simulink model "WormAndGearConstraint0x5B10x5D"  (R2024a)
settings: Solver=ode45  StartTime=0.0  StopTime=20  MaxStep=0.01  RelTol=1e-3
PreLoadFcn:
  | addpath(fullfile('WormAndGearConstraintSupport','Data'));
  | addpath(fullfile('WormAndGearConstraintSupport','Scripts'));
model workspace: external: MATLAB File WormAndGearConstraintParameters.m (data not in the file)
undefined symbols (not defined in the file): driveconn, frame, framemount, slewdrive, solarpanel, support, X, Y, Z
libraries: sm_lib x393, nesl_utility x10, fl_lib x4, SignalEditorBlockLib x2, fl_ps_legacy_lib x1
(part 1 of 11)
CloseFcn:
  | rmpath(fullfile('WormAndGearConstraintSupport','Data'));
  | rmpath(fullfile('WormAndGearConstraintSupport','Scripts'));
Description:
  | Using the Worm and Gear Constraint Block - Solar Tracker
settings Model: Creator=The MathWorks, Inc.  LastModifiedBy=Abhilash LN
settings SolverCC: AlgebraicLoopSolver=TrustRegion
settings OptimizationCC: ReuseModelBlockBuffer=off
settings DebuggingCC: UnconnectedInputMsg=warning  UnconnectedOutputMsg=warning  UnconnectedLineMsg=warning  SubsystemReferenceDiagnosticForUnitTest=warning  ArithmeticOperatorsInVariantConditions=warning
settings ModelReferenceCC: EnableRefExpFcnMdlSchedulingChecks=on
settings SFSimCC: SimUseLocalCustomCode=off  CustomCodeUndefinedFunction=UseInterfaceOnly
settings RTWCC: RTWUseLocalCustomCode=off  GPUComputeCapability=3.5
settings CodeAppCC: StateflowObjectComments=on
settings ConfigComp: CovMetricSettings=dswe
settings SimscapeCC: SimscapeNormalizeSystem=off  SimscapeNominalValues="[{\"value\":\"10\",\"unit\":\"V\"},{\"value\":\"1\",\"unit\":\"A\"},{\"value\":\"10\",\"unit\":\"N*m\"},{\"value\":\"10\",\"unit\":\"bar\"},{\"value\":\"100\",\"unit\":\"kJ/kg\"},{\"value\":\"1\",\"unit\":\"kW\"},{\"value\":\"300\",\"unit\":\"K\"},{\"value\":\"100\",\"unit\":\"cm^3/s\"},{\"value\":\"1\",\"unit\":\"kN\"},{\"value\":\"1\",\"unit\":\"g/cm^3\"},{\"value\":\"1\",\"unit\":\"l\"},{\"value\":\"1\",\"unit\":\"cm^2\"},{\"value\":\"60\",\"unit\":\"Hz\"}]"  SimscapeLogType=all  SimscapeLogSimulationStatistics=on  SimscapeLogName=simlogWormAndGearConstraint
settings DiagnosticsConfigSet: SimMechanicsUnconnectedFramePorts=none
settings ExplorerConfigSet: InternalSimMechanicsExplorerSettings="<ExplorerConfiguration><canonicalview>default</canonicalview><AnimationSetting><BasePlaybackSpeed>1.0</BasePlaybackSpeed><PlaybackSpeedFactor>1.0</PlaybackSpeedFactor></AnimationSetting><TilePanel><TileInfo><Tiles Columns=\"1\" Count=\"2\" Rows=\"2\"><Column Left=\"2\" Weight=\"1\"/><Column Left=\"959\" Weight=\"0.5003\"/><Row Top=\"2\" Weight=\"0.499\"/><Row Top=\"438\" Weight=\"0.501\"/><Row Top=\"875\"/><Tile Height=\"1\" Width=\"1\" X=\"0\" Y=\"0\"/><Tile Height=\"1\" Width=\"1\" X=\"0\" Y=\"1\"/></Tiles></TileInfo><SceneInfo><SceneViewer><BGColor><R>0.60000002384185791</R><G>0.60000002384185791</G><B>0.60000002384185791</B></BGColor><Camera><DoPerspective>off</DoPerspective><Position><X>1.5722270375482781</X><Y>0.036026125950558319</Y><Z>2.5132450829803226</Z></Position><Center><X>0.030597625568977493</X><Y>1.5776555379298589</Y><Z>0.97161567100102131</Z></Center><Up><X>-0.40824829046386307</X><Y>0.40824829046386307</Y><Z>0.81649658092772615</Z></Up><ViewLimDist>1</ViewLimDist><YLim>1.5517509961128235</YLim><XLim>3.445105256006924</XLim></Camera></SceneViewer><SceneViewer><BGColor><R>0.60000002384185791</R><G>0.60000002384185791</G><B>0.60000002384185791</B></BGColor><Camera><DoPerspective>on</DoPerspective><Position><X>0.052898448769590822</X><Y>3.2815089600888423</Y><Z>1.0106868675116196</Z></Position><Center><X>-0.01109217435380673</X><Y>3.0487464713239714</Y><Z>0.94979470185928261</Z></Center><Up><X>-0.054323829999052796</X><Y>-0.23871114009518463</Y><Z>0.96956996296744424</Z></Up><ViewLimDist>1</ViewLimDist><YLim>0.46630765815499858</YLim><XLim>1.0328496727358381</XLim></Camera></SceneViewer></SceneInfo></TilePanel><MechEditorPanel><Cameras><Camera><Id>Camera1</Id><Value><Name>Slew Drive View</Name><NativeCamera><PositionKeyframeSet><Keyframe><Time>+0.0000000000000000e+00</Time><Value><X>+5.2898448769590822e-02</X><Y>+3.2815089600888423e+00</Y><Z>+1.0106868675116196e+00</Z></Value></Keyframe></PositionKeyframeSet><CenterKeyframeSet><Keyframe><Time>+0.0000000000000000e+00</Time><Value><X>-1.1092174353806730e-02</X><Y>+3.0487464713239714e+00</Y><Z>+9.4979470185928261e-01</Z></Value></Keyframe></CenterKeyframeSet><UpVectorKeyframeSet><Keyframe><Time>+0.0000000000000000e+00</Time><Value><X>-5.4323829999052796e-02</X><Y>-2.3871114009518463e-01</Y><Z>+9.6956996296744424e-01</Z></Value></Keyframe></UpVectorKeyframeSet></NativeCamera></Value></Camera></Cameras><GfxPanelCameraMap><MapElement CameraMLId=\"Camera1\" GfxPanelIndex=\"1\"/></GfxPanelCameraMap><VideoCreator><PlaybackSpeedRatio>1.0</PlaybackSpeedRatio><FrameRate>30</FrameRate><VideoFormat>Motion JPEG AVI</VideoFormat><FrameSize>auto</FrameSize></VideoCreator></MechEditorPanel></ExplorerConfiguration>"

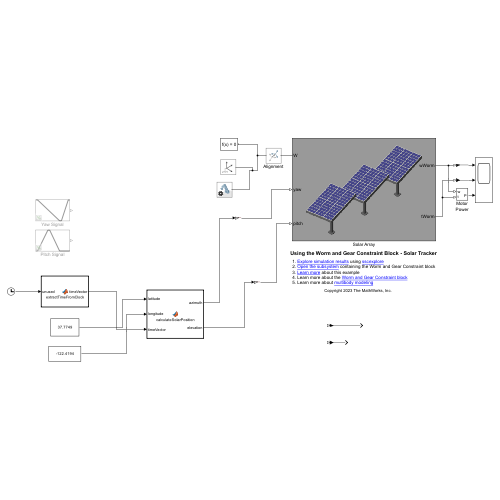
[thumbnail: Simulink's stored preview of the top-level diagram]
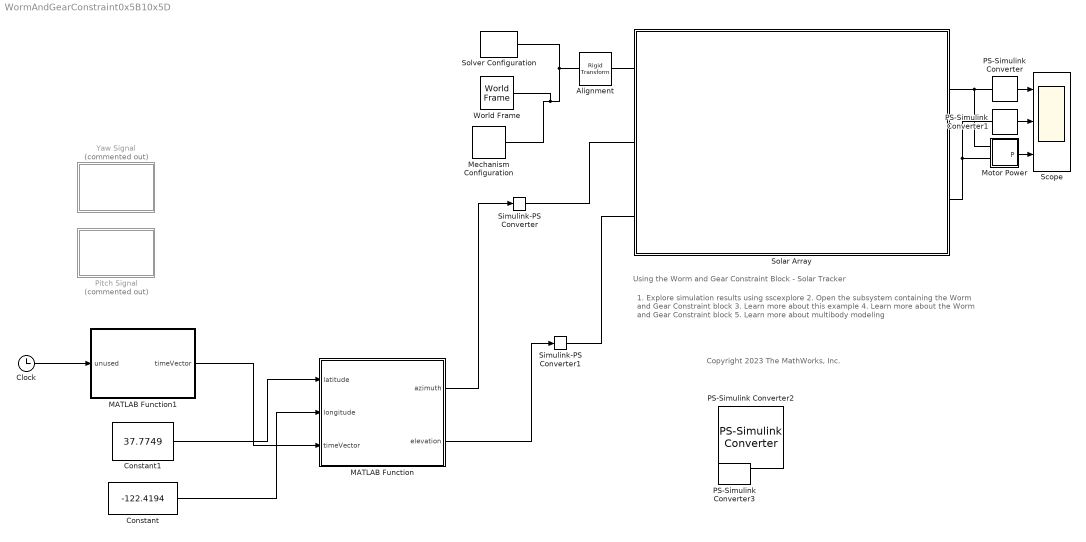
== system WormAndGearConstraint0x5B10x5D ==
  note: Copyright 2023 The MathWorks, Inc.
  note: Using the Worm and Gear Constraint Block - Solar Tracker
  note: 1. Explore simulation results using sscexplore
      | 2. Open the subsystem containing the Worm and Gear Constraint block
      | 3. Learn more about this example
      | 4. Learn more about the Worm and Gear Constraint block
      | 5. Learn more about multibody modeling
  Alignment : sm_lib/Frames and Transforms/Rigid Transform  RotationMethod=AlignedAxes  FollAlignAxisA=+Z  BaseAlignAxisA=+Z  FollAlignAxisB=+Y  BaseAlignAxisB=-X  RotationStandardAxis=+Z  RotationAngle=0.0  RotationAngleUnits=deg  RotationArbitraryAxis=[0 0 1]  RotationSequenceAxes=FollowerAxes  RotationSequence=XYX  RotationSequenceAngles=[0 0 0]  RotationSequenceAnglesUnits=deg  RotationMatrix=[1 0 0; 0 1 0; 0 0 1]  Quaternion=[1 0 0 0]  TranslationMethod=None  TranslationCartesianOffset=[0 0 0]  TranslationCartesianOffsetUnits=m  TranslationStandardAxis=+Z  TranslationStandardOffset=0  TranslationStandardOffsetUnits=m  TranslationROffset=0  TranslationROffsetUnits=m  TranslationThetaOffset=0  TranslationThetaOffsetUnits=deg  TranslationZOffset=0  TranslationZOffsetUnits=m
  Clock : Clock
  Constant : Constant  Value=-122.4194
  Constant1 : Constant  Value=37.7749
  MATLAB Function : MATLAB Function  TreatAsAtomicUnit=on
  MATLAB Function1 : MATLAB Function  TreatAsAtomicUnit=on
  Mechanism Configuration : sm_lib/Utilities/Mechanism Configuration  UniformGravity=Constant  GravityVector=[0 0 -9.80665]  GravityVectorUnits=m/s^2  LinearizationDelta=0.001  JointModeTransitionNonlinearIterations=2
  Motor Power : Subsystem
  PS-Simulink Converter : nesl_utility/PS-Simulink Converter  PhysicalDomain=network_engine_domain  SubClassName=ps_output  LeftPortType=input  RightPortType=output  PseudoPeriodic=off  Frequencies=[]  VectorFormat=1-D array  Unit=deg/s  AffineConversion=off
  PS-Simulink Converter1 : nesl_utility/PS-Simulink Converter  PhysicalDomain=network_engine_domain  SubClassName=ps_output  LeftPortType=input  RightPortType=output  PseudoPeriodic=off  Frequencies=[]  VectorFormat=1-D array  Unit=N*m  AffineConversion=off
  PS-Simulink Converter2 : nesl_utility/PS-Simulink Converter  PhysicalDomain=network_engine_domain  SubClassName=ps_output  LeftPortType=input  RightPortType=output  PseudoPeriodic=off  Frequencies=[]  VectorFormat=inherit  Unit=deg  AffineConversion=off
  PS-Simulink Converter3 : nesl_utility/PS-Simulink Converter  PhysicalDomain=network_engine_domain  SubClassName=ps_output  LeftPortType=input  RightPortType=output  PseudoPeriodic=off  Frequencies=[]  VectorFormat=inherit  Unit=deg  AffineConversion=off
  Pitch Signal : Subsystem  Commented=on
      mask Display: plot([0 1 7 8 14 20],[0 0 1 1 0 0])
  Scope : Scope  NumInputPorts=3
  Simulink-PS Converter : nesl_utility/Simulink-PS Converter  PhysicalDomain=network_engine_domain  SubClassName=ps_input  LeftPortType=input  RightPortType=output  PseudoPeriodic=off  Frequencies=[]  NoiseDistribution=none  NoiseParameters=[]  Unit=1  AffineConversion=off  FilteringAndDerivatives=provide  SimscapeFilterOrder=1  InputFilterTimeConstant=0.001  UdotUserProvided=0
  Simulink-PS Converter1 : nesl_utility/Simulink-PS Converter  PhysicalDomain=network_engine_domain  SubClassName=ps_input  LeftPortType=input  RightPortType=output  PseudoPeriodic=off  Frequencies=[]  NoiseDistribution=none  NoiseParameters=[]  Unit=1  AffineConversion=off  FilteringAndDerivatives=provide  SimscapeFilterOrder=1  InputFilterTimeConstant=0.001  UdotUserProvided=0
  Solar Array : Subsystem
      mask Display:
      | image(fullfile('WormAndGearConstraintSupport','Images','SolarArray.png'));
      | port_label('lconn',1,'W');
      | port_label('lconn',2,'yaw');
      | port_label('lconn',3,'pitch');
      | port_label('rconn',1,'wWorm');
      | port_label('rconn',2,'tWorm');
  Solver Configuration : nesl_utility/Solver Configuration  PhysicalDomain=network_engine_domain  SubClassName=solver  LeftPortType=input  RightPortType=generic  Tones=[]  Harmonics=[]  SimulateNoise=off  Profile=off  UseLocalSampling=off  EnableSwitchedLinearOptims=on  FrequencyDomain=off  UseCCode=off  RelTol=0.001  AbsTol=1e-06  MinStep=1e-09  ToWorkspace=off  RevertToSquareIcSolve=off  NumHomotopyIterations=100  PhasorMode=off  PhasorModeNumHarmonics=1  ConsistencySolver=NEWTON_XTOL_AFTER_FTOL  IndexReductionMethod=DerivativeReplacement  DoDC=off  ResidualTolerance=1e-09  ConsistencyTolSource=GLOBAL  ConsistencyAbsTol=0.001  ConsistencyRelTol=0.001  ConsistencyTolFactor=0.001  UseLocalSolver=off  LocalSolverChoice=NE_BACKWARD_EULER_ADVANCER  ResolveIndetEquations=on  FunctionEvalNumThread=1  LocalSolverSampleTime=0.001  DoFixedCost=off  MaxNonlinIter=3  MaxModeIter=2  ComputeImpulses=off  ImpulseIterations=2  LinearAlgebra=Sparse  LinearAlgebraNumThread=0  EquationFormulation=NE_TIME_EF  DelaysMemoryBudget=1024  AutomaticFiltering=on  FilteringTimeConstant=0.001  PartitionStorageMethod=AS_NEEDED  PartitionMemoryBudget=1024  PartitionMethod=FAST  MultibodyUseLocalSolver=off  MultibodyLocalSolverChoice=ODE1  MultibodyLocalSolverSampleTime=0.001
  World Frame : sm_lib/Frames and Transforms/World Frame
  Yaw Signal : Subsystem  Commented=on
      mask Display: plot([0 1 14 15 19 20], [0 0 -1 -1 0 0])
  wires:
  PS-Simulink Converter1/1 -> Scope/2
  PS-Simulink Converter/1 -> Scope/1
  Motor Power/1(P) -> Scope/3
  Constant/1 -> MATLAB Function/2(longitude)
  MATLAB Function1/1(timeVector) -> MATLAB Function/3(timeVector)
  Clock/1 -> MATLAB Function1/1(unused)
  Constant1/1 -> MATLAB Function/1(latitude)
  MATLAB Function/2(elevation) -> Simulink-PS Converter1/1
  MATLAB Function/1(azimuth) -> Simulink-PS Converter/1
  connections:
  World Frame/RConn1 -- Solver Configuration/RConn1 -- Alignment/LConn1 -- Mechanism Configuration/RConn1
  Alignment/RConn1 -- Solar Array/LConn1
  PS-Simulink Converter/LConn1 -- Motor Power/LConn1 -- Solar Array/RConn1
  PS-Simulink Converter1/LConn1 -- Motor Power/LConn2 -- Solar Array/RConn2
  Simulink-PS Converter/RConn1 -- Solar Array/LConn2
  Simulink-PS Converter1/RConn1 -- Solar Array/LConn3

== system WormAndGearConstraint0x5B10x5D/Motor Power ==
  Motor Power : fl_ps_legacy_lib/Legacy Physical Signals/Functions/PS Product
  PS-Simulink Converter2 : nesl_utility/PS-Simulink Converter  PhysicalDomain=network_engine_domain  SubClassName=ps_output  LeftPortType=input  RightPortType=output  PseudoPeriodic=off  Frequencies=[]  VectorFormat=1-D array  Unit=kW  AffineConversion=off
  w : PMIOPort  Side=Left
  t : PMIOPort  Port=2  Side=Left
  P : Outport
  wires:
  PS-Simulink Converter2/1 -> P/1
  connections:
  PS-Simulink Converter2/LConn1 -- Motor Power/RConn1
  Motor Power/LConn2 -- t/RConn1
  Motor Power/LConn1 -- w/RConn1

== system WormAndGearConstraint0x5B10x5D/Pitch Signal ==
  Pitch Signal : SignalEditorBlockLib/Signal Editor  FileName=WormAndGearConstraintInput2.mat  ActiveScenario=Group_1  ActiveSignal=Signal 2  IsBus=off  OutputBusObjectStr=Bus: BusObject  SampleTime=0  OutputAfterFinalValue=Extrapolation  Unit=inherit  PreserveSignalName=on  ApplySigPropsToAllScenarios=on  ApplySigPropsToAllSignals=off
  Simulink-PS Converter2 : nesl_utility/Simulink-PS Converter  PhysicalDomain=network_engine_domain  SubClassName=ps_input  LeftPortType=input  RightPortType=output  PseudoPeriodic=off  Frequencies=[]  NoiseDistribution=none  NoiseParameters=[]  Unit=deg  AffineConversion=off  FilteringAndDerivatives=filter  SimscapeFilterOrder=2  InputFilterTimeConstant=pitchsignal.t_c  UdotUserProvided=1
  Signal : PMIOPort  Side=Right
  wires:
  Pitch Signal/1 -> Simulink-PS Converter2/1
  connections:
  Signal/RConn1 -- Simulink-PS Converter2/RConn1

== system WormAndGearConstraint0x5B10x5D/Solar Array ==
  Solar Tracker1 : Subsystem
      mask Display:
      | image(fullfile('WormAndGearConstraintSupport','Images','SolarTracker.png'));
      | port_label('lconn',1,'B');
      | port_label('lconn',2,'y');
      | port_label('lconn',3,'p');
  Solar Tracker2 : Subsystem
      mask Display:
      | image(fullfile('WormAndGearConstraintSupport','Images','SolarTracker.png'));
      | port_label('lconn',1,'B');
      | port_label('lconn',2,'y');
      | port_label('lconn',3,'p');
  Solar Tracker3 : Subsystem
      mask Display:
      | image(fullfile('WormAndGearConstraintSupport','Images','SolarTracker.png'));
      | port_label('lconn',1,'B');
      | port_label('lconn',2,'y');
      | port_label('lconn',3,'p');
      | port_label('rconn',1,'w');
      | port_label('rconn',2,'t');
  Tracker1 xForm : sm_lib/Frames and Transforms/Rigid Transform  RotationMethod=None  FollAlignAxisA=+X  BaseAlignAxisA=+Y  FollAlignAxisB=+Y  BaseAlignAxisB=+Z  RotationStandardAxis=+Z  RotationAngle=0.0  RotationAngleUnits=deg  RotationArbitraryAxis=[0 0 1]  RotationSequenceAxes=FollowerAxes  RotationSequence=XYX  RotationSequenceAngles=[0 0 0]  RotationSequenceAnglesUnits=deg  RotationMatrix=[1 0 0; 0 1 0; 0 0 1]  Quaternion=[1 0 0 0]  TranslationMethod=Cartesian  TranslationCartesianOffset=tracker1_offset  TranslationCartesianOffsetUnits=m  TranslationStandardAxis=+Z  TranslationStandardOffset=0  TranslationStandardOffsetUnits=m  TranslationROffset=0  TranslationROffsetUnits=m  TranslationThetaOffset=0  TranslationThetaOffsetUnits=deg  TranslationZOffset=0  TranslationZOffsetUnits=m
  Tracker2 xForm : sm_lib/Frames and Transforms/Rigid Transform  RotationMethod=None  FollAlignAxisA=+Z  BaseAlignAxisA=+Z  FollAlignAxisB=+Y  BaseAlignAxisB=-X  RotationStandardAxis=+Z  RotationAngle=0.0  RotationAngleUnits=deg  RotationArbitraryAxis=[0 0 1]  RotationSequenceAxes=FollowerAxes  RotationSequence=XYX  RotationSequenceAngles=[0 0 0]  RotationSequenceAnglesUnits=deg  RotationMatrix=[1 0 0; 0 1 0; 0 0 1]  Quaternion=[1 0 0 0]  TranslationMethod=Cartesian  TranslationCartesianOffset=tracker2_offset  TranslationCartesianOffsetUnits=m  TranslationStandardAxis=+Z  TranslationStandardOffset=0  TranslationStandardOffsetUnits=m  TranslationROffset=0  TranslationROffsetUnits=m  TranslationThetaOffset=0  TranslationThetaOffsetUnits=deg  TranslationZOffset=0  TranslationZOffsetUnits=m
  Tracker3 xForm : sm_lib/Frames and Transforms/Rigid Transform  RotationMethod=None  FollAlignAxisA=+X  BaseAlignAxisA=+Y  FollAlignAxisB=+Y  BaseAlignAxisB=+Z  RotationStandardAxis=+Z  RotationAngle=0.0  RotationAngleUnits=deg  RotationArbitraryAxis=[0 0 1]  RotationSequenceAxes=FollowerAxes  RotationSequence=XYX  RotationSequenceAngles=[0 0 0]  RotationSequenceAnglesUnits=deg  RotationMatrix=[1 0 0; 0 1 0; 0 0 1]  Quaternion=[1 0 0 0]  TranslationMethod=Cartesian  TranslationCartesianOffset=tracker3_offset  TranslationCartesianOffsetUnits=m  TranslationStandardAxis=+Z  TranslationStandardOffset=0  TranslationStandardOffsetUnits=m  TranslationROffset=0  TranslationROffsetUnits=m  TranslationThetaOffset=0  TranslationThetaOffsetUnits=deg  TranslationZOffset=0  TranslationZOffsetUnits=m
  W : PMIOPort  Side=Left
  wWorm : PMIOPort  Port=2  Side=Right
  yaw : PMIOPort  Port=3  Side=Left
  tWorm : PMIOPort  Port=4  Side=Right
  pitch : PMIOPort  Port=5  Side=Left
  connections:
  Tracker3 xForm/LConn1 -- Tracker1 xForm/LConn1 -- W/RConn1 -- Tracker2 xForm/LConn1
  Tracker3 xForm/RConn1 -- Solar Tracker3/LConn1
  Solar Tracker3/RConn2 -- tWorm/RConn1
  Solar Tracker3/LConn3 -- Solar Tracker2/LConn3 -- Solar Tracker1/LConn3 -- pitch/RConn1
  Solar Tracker3/RConn1 -- wWorm/RConn1
  Solar Tracker2/LConn2 -- Solar Tracker1/LConn2 -- Solar Tracker3/LConn2 -- yaw/RConn1
  Tracker2 xForm/RConn1 -- Solar Tracker2/LConn1
  Tracker1 xForm/RConn1 -- Solar Tracker1/LConn1

== system WormAndGearConstraint0x5B10x5D/Yaw Signal ==
  Simulink-PS Converter1 : nesl_utility/Simulink-PS Converter  PhysicalDomain=network_engine_domain  SubClassName=ps_input  LeftPortType=input  RightPortType=output  PseudoPeriodic=off  Frequencies=[]  NoiseDistribution=none  NoiseParameters=[]  Unit=deg  AffineConversion=off  FilteringAndDerivatives=filter  SimscapeFilterOrder=2  InputFilterTimeConstant=yawsignal.t_c  UdotUserProvided=1
  Yaw Signal : SignalEditorBlockLib/Signal Editor  FileName=WormAndGearConstraintInput1.mat  ActiveScenario=Group_1  ActiveSignal=Signal  IsBus=off  OutputBusObjectStr=Bus: BusObject  SampleTime=0  Interpolate=off  ZeroCross=off  OutputAfterFinalValue=Setting to zero  Unit=inherit  PreserveSignalName=on  ApplySigPropsToAllScenarios=on  ApplySigPropsToAllSignals=off
  Signal : PMIOPort  Side=Right
  wires:
  Yaw Signal/1 -> Simulink-PS Converter1/1
  connections:
  Signal/RConn1 -- Simulink-PS Converter1/RConn1

== system WormAndGearConstraint0x5B10x5D/Solar Array/Solar Tracker1 ==
  Drive Connection : Subsystem  AncestorBlock=WormAndGearConstraintLibrary/Drive Connection  mask(Drive Connection){connRadius=driveconn.connectionRadius, connThickness=driveconn.connectionThickness, connLength=driveconn.connectionLength, bracketWidth=driveconn.bracketWidthHeight, bracketThickness=driveconn.bracketThickness, holeRadius=driveconn.holeRadius, holeOffset=driveconn.holeOffset, baseThickness=driveconn.baseThickness, rho=driveconn.density, color=driveconn.color}
      mask prompts: connRadius "Connection Radius (m)"; connThickness "Connection Thickness (m)"; connLength "Connection Length (m)"; bracketWidth "Bracket Width and Height (m)"; bracketThickness "Bracket Thickness (m)"; holeRadius "Hole Radius (m)"; holeOffset "Hole Offset (m)"; baseThickness "Base Thickness (m)"; rho "Density (kg/m^3)"; color "Color [r g b]"
      mask help:
      | This block models the element that connects the solar array assembly to the slew drive.
      |
      | Port B corresponds to the center of the base face of the drive connection. Port H corresponds to the center of the bracket hole.
      mask init:
      | baseAngle = atan(bracketWidth / bracketThickness);
      | baseRadius = 0.5 * bracketThickness / cos(baseAngle);
      settings: LibrarySourceBlock=sm_solar_tracker_lib/Drive Connection
      mask DialogControl Tab1 Prompt: Dimensions
      mask DialogControl Tab2 Prompt: Material Properties
      mask Display:
      | image(fullfile('WormAndGearConstraintSupport','Images','DriveConnection.png'));
      | port_label('lconn',1,'B');
      | port_label('rconn',1,'H');
  PS Terminator : fl_lib/Physical Signals/Sinks/PS Terminator
  PS Terminator1 : fl_lib/Physical Signals/Sinks/PS Terminator
  Panel Revolute : sm_lib/Joints/Revolute Joint  JointMode=Normal  CompositeWrenchDir=FollowerOnBase  CompositeWrenchFrame=BaseFrame  SenseConstraintForce=off  SenseConstraintTorque=off  SenseTotalForce=off  SenseTotalTorque=off  PositionTargetSpecify=on  PositionTargetPriority=High  PositionTargetValue=panelrevolute.q0  PositionTargetValueUnits=deg  VelocityTargetSpecify=off  VelocityTargetPriority=High  VelocityTargetValue=0  VelocityTargetValueUnits=deg/s  EquilibriumPosition=0  EquilibriumPositionUnits=deg  SpringStiffness=0  SpringStiffnessUnits=N*m/deg  DampingCoefficient=0  DampingCoefficientUnits=N*m/(deg/s)  LowerLimitSpecify=off  LowerLimitBound=-90  LowerLimitBoundUnits=deg  LowerLimitStiffness=1e4  LowerLimitStiffnessUnits=N*m/deg  LowerLimitDamping=10  LowerLimitDampingUnits=N*m/(deg/s)  LowerLimitTransitionRegionWidth=0.1  LowerLimitTransitionRegionWidthUnits=deg  UpperLimitSpecify=off  UpperLimitBound=90  UpperLimitBoundUnits=deg  UpperLimitStiffness=1e4  UpperLimitStiffnessUnits=N*m/deg  UpperLimitDamping=10  UpperLimitDampingUnits=N*m/(deg/s)  UpperLimitTransitionRegionWidth=0.1  UpperLimitTransitionRegionWidthUnits=deg  TorqueActuationMode=ComputedTorque  MotionActuationMode=InputMotion  SensePosition=off  SenseVelocity=off  SenseAcceleration=off  SenseTorqueForce=off  SenseLowerLimitTorqueForce=off  SenseUpperLimitTorqueForce=off
  Slew Drive : Subsystem  AncestorBlock=WormAndGearConstraintLibrary/Slew Drive  mask(Slew Drive){wormLeadAngle=slewdrive.wormLeadAngle, wormLength=slewdrive.wormLength, gearOuterRadius=slewdrive.gearOuterRadius, gearInnerRadius=slewdrive.gearInnerRadius, gearExposedRadius=slewdrive.gearExposedRadius, ratio=slewdrive.ratio, housingThickness=slewdrive.housingThickness, bWormRevolute=slewdrive.wormRevoluteDamping, wormRho=slewdrive.wormDensity, gearRho=slewdrive.gearDensity, housingRho=slewdrive.housingDensity, wormColor=slewdrive.wormColor, gearColor=slewdrive.gearColor, housingColor=slewdrive.housingColor, housingOpacity=slewdrive.housingOpacity}
      mask prompts: wormLeadAngle "Worm Lead Angle (deg)"; wormLength "Worm Length (m)"; gearOuterRadius "Gear Outer Radius (m)"; gearInnerRadius "Gear Inner Radius (m)"; gearExposedRadius "Gear Exposed Radius (m)"; ratio "Ratio (Ng / Nw)"; housingThickness "Housing Thickness (m)"; bWormRevolute "Worm Revolute Damping (Nm/(deg/s))"; wormRho "Worm Density (kg/m^3)"; gearRho "Gear Density (kg/m^3)"; housingRho "Housing Density (kg/m3)"; wormColor "Worm Color [r g b]"; gearColor "Gear Color [r g b]"; housingColor "Housing Color [r g b]"; housingOpacity "Housing Opacity"
      mask help:
      | This block models the slew drive of the solar tracker.
      |
      | Port B corresponds to the base face of the housing aligned with the gear axis. Port T corresponds to the center of the top face of the gear.
      |
      | Input port q specifies the motion actuation signal of the gear revolute. Output port w corresponds to the angular velocity of the worm revolute. Output port t corresponds to the automatically computed actuation torque at the worm revolute necessary to achieve the desired motion signal of the gear revolute.
      mask init:
      | % Worm Properties
      | wormRadius            = gearOuterRadius / (ratio * tand(wormLeadAngle));
      | wormNonThreadedRadius = 0.4*wormRadius;
      | 
      | wormThreadedLength    = 0.4*wormLength;
      | wormNonThreadedLength = 0.5*(wormLength - wormThreadedLength);
      | 
      | wormHoleRadius = 0.5*wormNonThreadedRadius;
      | 
      | wormThreadedThickness    = wormRadius - wormHoleRadius;
      | wormNonThreadedThickness = wormNonThreadedRadius - wormHoleRadius;
      | 
      | wormSliceColor      = 0.75*wormColor;
      | wormSliceProportion = 0.25;
      | 
      | % Worm Offsets
      | wormLeftOffset  = [-0.5*wormLength gearOuterRadius+wormRadius 0];
      | wormRightOffset = [ 0.5*wormLength gearOuterRadius+wormRadius 0];
      | 
      | % Gear Properties
      | gearLength         = wormRadius;
      | gearThickness      = gearOuterRadius - gearInnerRadius;
      | gearSliceThickness = 0.1*gearOuterRadius;
      | gearSliceColor     = 0.75*gearColor;
      | 
      | % Housing Dimensions
      | housingRadTol = 0.05*gearOuterRadius;
      | sideDepth     = 2*wormRadius + 2*housingRadTol;
      | 
      | % Housing Base Vertices
      | baseVertex1_x = 0;
      | baseVertex2_x = housingThickness + housingRadTol + 2*wormRadius;
      | baseVertex3_x = baseVertex2_x + gearOuterRadius;
      | baseVertex4_x = baseVertex3_x + gearOuterRadius + housingRadTol + housingThickness;
      | 
      | baseVertex1_y = -0.5*wormLength - housingThickness;
      | baseVertex2_y = baseVertex1_y;
      | baseVertex3_y = -gearOuterRadius - housingRadTol - housingThickness;
      | baseVertex4_y = baseVertex3_y;
      | 
      | baseVertices = [...
      |   baseVertex1_x  baseVertex1_y;...
      |   baseVertex2_x  baseVertex2_y;...
      |   baseVertex3_x  baseVertex3_y;...
      |   baseVertex4_x  baseVertex4_y;...
      |   baseVertex4_x -baseVertex4_y;...
      |   baseVertex3_x -baseVertex3_y;...
      |   baseVertex2_x -baseVertex2_y;...
      |   baseVertex1_x -baseVertex1_y];
      | 
      | baseVertex1_R = 0.5*wormRadius + housingRadTol + housingThickness;
      | baseVertex4_R = gearOuterRadius + housingRadTol + housingThickness;
      | baseVertex5_R = baseVertex4_R;
      | baseVertex8_R = baseVertex1_R;
      | 
      | baseVerticesR = [baseVertex1_R baseVertex4_R baseVertex5_R baseVertex8_R];
      |   
      | baseVertices = simmechanics.demohelpers.round_corners(...
      |   baseVertices, [1 4 5 8], baseVerticesR, 20);
      | 
      | % Housing Side Vertices
      | sideVertices = [...
      |   baseVertex1_x+housingThickness  baseVertex1_y+housingThickness;...
      |   baseVertex2_x                   baseVertex2_y+housingThickness;...
      |   baseVertex3_x                   baseVertex3_y+housingThickness;...
      |   baseVertex4_x-housingThickness  baseVertex4_y+housingThickness;...
      |   baseVertex4_x-housingThickness -baseVertex4_y-housingThickness;...
      |   baseVertex3_x                  -baseVertex3_y-housingThickness;...
      |   baseVertex2_x                  -baseVertex2_y-housingThickness;...
      |   baseVertex1_x+housingThickness -baseVertex1_y-housingThickness];
      | 
      | sideVertex1_R = 0.5*wormRadius + housingRadTol;
      | sideVertex4_R = gearOuterRadius + housingRadTol;
      | sideVertex5_R = sideVertex4_R;
      | sideVertex8_R = sideVertex1_R;
      | 
      | sideVerticesR = [sideVertex1_R sideVertex4_R sideVertex5_R sideVertex8_R];
      | 
      | sideVertices = simmechanics.demohelpers.round_corners(...
      |   sideVertices, [1 4 5 8], sideVerticesR, 20);
      | 
      | sideVertices = flipud(sideVertices);
      | sideVertices(end+1,:) = sideVertices(1,:);
      | 
      | sideVertices = [sideVertices; baseVertices(end,:); baseVertices];
      | 
      | % Housing Top Vertices
      | topHoleOffset = housingThickness + housingRadTol + 2*wormRadius + gearOuterRadius;
      | 
      | topHoleTheta = linspace(pi, -pi, 40);
      | topVertices = [gearExposedRadius*cos(topHoleTheta)+topHoleOffset;...
      |                gearExposedRadius*sin(topHoleTheta)]';
      | 
      | topVertices = [topVertices; 0 0; baseVertices; 0 0];
      | 
      | % Housing Offsets
      | housingOffset        = topHoleOffset;
      | housingTopBaseOffset = 0.5*sideDepth + 0.5*housingThickness;
      | baseOffset           = [topHoleOffset 0 -0.5*housingThickness];
      settings: LibrarySourceBlock=sm_solar_tracker_lib/Slew Drive
      mask DialogControl Tab1 Prompt: Dimensions
      mask DialogControl Tab2 Prompt: Internal Mechanics
      mask DialogControl Tab3 Prompt: Material Properties
      mask Display:
      | image(fullfile('WormAndGearConstraintSupport','Images','SlewDrive.png'));
      | port_label('lconn',1,'B');
      | port_label('lconn',2,'q');
      | port_label('rconn',1,'T');
      | port_label('rconn',2,'w');
      | port_label('rconn',3,'t');
  Solar Panel Assembly : Subsystem
      mask Display:
      | image(fullfile('WormAndGearConstraintSupport','Images','SolarPanel.png'));
      | port_label('lconn',1,'H');
  Support : Subsystem  AncestorBlock=WormAndGearConstraintLibrary/Support  mask(Support){columnRadius=support.columnRadius, columnThickness=support.columnThickness, columnHeight=support.columnHeight, baseWidth=support.baseWidth, baseThickness=support.baseThickness, rho=support.density, color=support.color}
      mask prompts: columnRadius "Column Radius (m)"; columnThickness "Column Thickness (m)"; columnHeight "Column Height (m)"; baseWidth "Base Width (m)"; baseThickness "Base Thickness (m)"; rho "Density (kg/m^3)"; color "Color [r g b]"
      mask help:
      | This block models the support for the solar tracker.
      |
      | Port B corresponds to the center of the base face. Port T corresponds to the center of the top face of the column.
      mask init:
      | halfBaseWidth = 0.5*baseWidth;
      | 
      | baseVertices = [...
      |   -halfBaseWidth -halfBaseWidth;...
      |    halfBaseWidth -halfBaseWidth;...
      |    halfBaseWidth  halfBaseWidth;...
      |   -halfBaseWidth  halfBaseWidth];
      | 
      | baseVertices = simmechanics.demohelpers.round_corners(...
      |   baseVertices, [1:4], 0.5*halfBaseWidth, 10);
      settings: LibrarySourceBlock=sm_solar_tracker_lib/Support
      mask DialogControl Tab1 Prompt: Dimensions
      mask DialogControl Tab2 Prompt: Material Properties
      mask Display:
      | image(fullfile('WormAndGearConstraintSupport','Images','Support.png'));
      | port_label('lconn',1,'B');
      | port_label('rconn',1,'T');
  B : PMIOPort  Side=Left
  y : PMIOPort  Port=2  Side=Left
  p : PMIOPort  Port=3  Side=Left
  connections:
  Support/LConn1 -- B/RConn1
  Support/RConn1 -- Slew Drive/LConn1
  Drive Connection/LConn1 -- Slew Drive/RConn1
  Panel Revolute/LConn1 -- Drive Connection/RConn1
  PS Terminator/LConn1 -- Slew Drive/RConn2
  Slew Drive/LConn2 -- y/RConn1
  Panel Revolute/LConn2 -- p/RConn1
  Panel Revolute/RConn1 -- Solar Panel Assembly/LConn1
  PS Terminator1/LConn1 -- Slew Drive/RConn3

== system WormAndGearConstraint0x5B10x5D/Solar Array/Solar Tracker2 ==
  Drive Connection : Subsystem  AncestorBlock=WormAndGearConstraintLibrary/Drive Connection  mask(Drive Connection){connRadius=driveconn.connectionRadius, connThickness=driveconn.connectionThickness, connLength=driveconn.connectionLength, bracketWidth=driveconn.bracketWidthHeight, bracketThickness=driveconn.bracketThickness, holeRadius=driveconn.holeRadius, holeOffset=driveconn.holeOffset, baseThickness=driveconn.baseThickness, rho=driveconn.density, color=driveconn.color}
      mask prompts: connRadius "Connection Radius (m)"; connThickness "Connection Thickness (m)"; connLength "Connection Length (m)"; bracketWidth "Bracket Width and Height (m)"; bracketThickness "Bracket Thickness (m)"; holeRadius "Hole Radius (m)"; holeOffset "Hole Offset (m)"; baseThickness "Base Thickness (m)"; rho "Density (kg/m^3)"; color "Color [r g b]"
      mask help:
      | This block models the element that connects the solar array assembly to the slew drive.
      |
      | Port B corresponds to the center of the base face of the drive connection. Port H corresponds to the center of the bracket hole.
      mask init:
      | baseAngle = atan(bracketWidth / bracketThickness);
      | baseRadius = 0.5 * bracketThickness / cos(baseAngle);
      settings: LibrarySourceBlock=sm_solar_tracker_lib/Drive Connection
      mask DialogControl Tab1 Prompt: Dimensions
      mask DialogControl Tab2 Prompt: Material Properties
      mask Display:
      | image(fullfile('WormAndGearConstraintSupport','Images','DriveConnection.png'));
      | port_label('lconn',1,'B');
      | port_label('rconn',1,'H');
  PS Terminator : fl_lib/Physical Signals/Sinks/PS Terminator
  PS Terminator1 : fl_lib/Physical Signals/Sinks/PS Terminator
  Panel Revolute : sm_lib/Joints/Revolute Joint  JointMode=Normal  CompositeWrenchDir=FollowerOnBase  CompositeWrenchFrame=BaseFrame  SenseConstraintForce=off  SenseConstraintTorque=off  SenseTotalForce=off  SenseTotalTorque=off  PositionTargetSpecify=on  PositionTargetPriority=High  PositionTargetValue=panelrevolute.q0  PositionTargetValueUnits=deg  VelocityTargetSpecify=off  VelocityTargetPriority=High  VelocityTargetValue=0  VelocityTargetValueUnits=deg/s  EquilibriumPosition=0  EquilibriumPositionUnits=deg  SpringStiffness=0  SpringStiffnessUnits=N*m/deg  DampingCoefficient=0  DampingCoefficientUnits=N*m/(deg/s)  LowerLimitSpecify=off  LowerLimitBound=-90  LowerLimitBoundUnits=deg  LowerLimitStiffness=1e4  LowerLimitStiffnessUnits=N*m/deg  LowerLimitDamping=10  LowerLimitDampingUnits=N*m/(deg/s)  LowerLimitTransitionRegionWidth=0.1  LowerLimitTransitionRegionWidthUnits=deg  UpperLimitSpecify=off  UpperLimitBound=90  UpperLimitBoundUnits=deg  UpperLimitStiffness=1e4  UpperLimitStiffnessUnits=N*m/deg  UpperLimitDamping=10  UpperLimitDampingUnits=N*m/(deg/s)  UpperLimitTransitionRegionWidth=0.1  UpperLimitTransitionRegionWidthUnits=deg  TorqueActuationMode=ComputedTorque  MotionActuationMode=InputMotion  SensePosition=off  SenseVelocity=off  SenseAcceleration=off  SenseTorqueForce=off  SenseLowerLimitTorqueForce=off  SenseUpperLimitTorqueForce=off
  Slew Drive : Subsystem  AncestorBlock=WormAndGearConstraintLibrary/Slew Drive  mask(Slew Drive){wormLeadAngle=slewdrive.wormLeadAngle, wormLength=slewdrive.wormLength, gearOuterRadius=slewdrive.gearOuterRadius, gearInnerRadius=slewdrive.gearInnerRadius, gearExposedRadius=slewdrive.gearExposedRadius, ratio=slewdrive.ratio, housingThickness=slewdrive.housingThickness, bWormRevolute=slewdrive.wormRevoluteDamping, wormRho=slewdrive.wormDensity, gearRho=slewdrive.gearDensity, housingRho=slewdrive.housingDensity, wormColor=slewdrive.wormColor, gearColor=slewdrive.gearColor, housingColor=slewdrive.housingColor, housingOpacity=slewdrive.housingOpacity}
      mask prompts: wormLeadAngle "Worm Lead Angle (deg)"; wormLength "Worm Length (m)"; gearOuterRadius "Gear Outer Radius (m)"; gearInnerRadius "Gear Inner Radius (m)"; gearExposedRadius "Gear Exposed Radius (m)"; ratio "Ratio (Ng / Nw)"; housingThickness "Housing Thickness (m)"; bWormRevolute "Worm Revolute Damping (Nm/(deg/s))"; wormRho "Worm Density (kg/m^3)"; gearRho "Gear Density (kg/m^3)"; housingRho "Housing Density (kg/m3)"; wormColor "Worm Color [r g b]"; gearColor "Gear Color [r g b]"; housingColor "Housing Color [r g b]"; housingOpacity "Housing Opacity"
      mask help:
      | This block models the slew drive of the solar tracker.
      |
      | Port B corresponds to the base face of the housing aligned with the gear axis. Port T corresponds to the center of the top face of the gear.
      |
      | Input port q specifies the motion actuation signal of the gear revolute. Output port w corresponds to the angular velocity of the worm revolute. Output port t corresponds to the automatically computed actuation torque at the worm revolute necessary to achieve the desired motion signal of the gear revolute.
      mask init: same as WormAndGearConstraint0x5B10x5D/Solar Array/Solar Tracker1/Slew Drive
      settings: LibrarySourceBlock=sm_solar_tracker_lib/Slew Drive
      mask DialogControl Tab1 Prompt: Dimensions
      mask DialogControl Tab2 Prompt: Internal Mechanics
      mask DialogControl Tab3 Prompt: Material Properties
      mask Display:
      | image(fullfile('WormAndGearConstraintSupport','Images','SlewDrive.png'));
      | port_label('lconn',1,'B');
      | port_label('lconn',2,'q');
      | port_label('rconn',1,'T');
      | port_label('rconn',2,'w');
      | port_label('rconn',3,'t');
  Solar Panel Assembly : Subsystem
      mask Display:
      | image(fullfile('WormAndGearConstraintSupport','Images','SolarPanel.png'));
      | port_label('lconn',1,'H');
  Support : Subsystem  AncestorBlock=WormAndGearConstraintLibrary/Support  mask(Support){columnRadius=support.columnRadius, columnThickness=support.columnThickness, columnHeight=support.columnHeight, baseWidth=support.baseWidth, baseThickness=support.baseThickness, rho=support.density, color=support.color}
      mask prompts: columnRadius "Column Radius (m)"; columnThickness "Column Thickness (m)"; columnHeight "Column Height (m)"; baseWidth "Base Width (m)"; baseThickness "Base Thickness (m)"; rho "Density (kg/m^3)"; color "Color [r g b]"
      mask help:
      | This block models the support for the solar tracker.
      |
      | Port B corresponds to the center of the base face. Port T corresponds to the center of the top face of the column.
      mask init: same as WormAndGearConstraint0x5B10x5D/Solar Array/Solar Tracker1/Support
      settings: LibrarySourceBlock=sm_solar_tracker_lib/Support
      mask DialogControl Tab1 Prompt: Dimensions
      mask DialogControl Tab2 Prompt: Material Properties
      mask Display:
      | image(fullfile('WormAndGearConstraintSupport','Images','Support.png'));
      | port_label('lconn',1,'B');
      | port_label('rconn',1,'T');
  B : PMIOPort  Side=Left
  y : PMIOPort  Port=2  Side=Left
  p : PMIOPort  Port=3  Side=Left
  connections:
  PS Terminator1/LConn1 -- Slew Drive/RConn3
  Panel Revolute/RConn1 -- Solar Panel Assembly/LConn1
  Panel Revolute/LConn2 -- p/RConn1
  Slew Drive/LConn2 -- y/RConn1
  PS Terminator/LConn1 -- Slew Drive/RConn2
  Panel Revolute/LConn1 -- Drive Connection/RConn1
  Drive Connection/LConn1 -- Slew Drive/RConn1
  Support/RConn1 -- Slew Drive/LConn1
  Support/LConn1 -- B/RConn1

== system WormAndGearConstraint0x5B10x5D/Solar Array/Solar Tracker3 ==
  Drive Connection : Subsystem  AncestorBlock=WormAndGearConstraintLibrary/Drive Connection  mask(Drive Connection){connRadius=driveconn.connectionRadius, connThickness=driveconn.connectionThickness, connLength=driveconn.connectionLength, bracketWidth=driveconn.bracketWidthHeight, bracketThickness=driveconn.bracketThickness, holeRadius=driveconn.holeRadius, holeOffset=driveconn.holeOffset, baseThickness=driveconn.baseThickness, rho=driveconn.density, color=driveconn.color}
      mask prompts: connRadius "Connection Radius (m)"; connThickness "Connection Thickness (m)"; connLength "Connection Length (m)"; bracketWidth "Bracket Width and Height (m)"; bracketThickness "Bracket Thickness (m)"; holeRadius "Hole Radius (m)"; holeOffset "Hole Offset (m)"; baseThickness "Base Thickness (m)"; rho "Density (kg/m^3)"; color "Color [r g b]"
      mask help:
      | This block models the element that connects the solar array assembly to the slew drive.
      |
      | Port B corresponds to the center of the base face of the drive connection. Port H corresponds to the center of the bracket hole.
      mask init:
      | baseAngle = atan(bracketWidth / bracketThickness);
      | baseRadius = 0.5 * bracketThickness / cos(baseAngle);
      settings: LibrarySourceBlock=sm_solar_tracker_lib/Drive Connection
      mask DialogControl Tab1 Prompt: Dimensions
      mask DialogControl Tab2 Prompt: Material Properties
      mask Display:
      | image(fullfile('WormAndGearConstraintSupport','Images','DriveConnection.png'));
      | port_label('lconn',1,'B');
      | port_label('rconn',1,'H');
  Panel Revolute : sm_lib/Joints/Revolute Joint  JointMode=Normal  CompositeWrenchDir=FollowerOnBase  CompositeWrenchFrame=BaseFrame  SenseConstraintForce=off  SenseConstraintTorque=off  SenseTotalForce=off  SenseTotalTorque=off  PositionTargetSpecify=on  PositionTargetPriority=High  PositionTargetValue=panelrevolute.q0  PositionTargetValueUnits=deg  VelocityTargetSpecify=off  VelocityTargetPriority=High  VelocityTargetValue=0  VelocityTargetValueUnits=deg/s  EquilibriumPosition=0  EquilibriumPositionUnits=deg  SpringStiffness=0  SpringStiffnessUnits=N*m/deg  DampingCoefficient=0  DampingCoefficientUnits=N*m/(deg/s)  LowerLimitSpecify=off  LowerLimitBound=-90  LowerLimitBoundUnits=deg  LowerLimitStiffness=1e4  LowerLimitStiffnessUnits=N*m/deg  LowerLimitDamping=10  LowerLimitDampingUnits=N*m/(deg/s)  LowerLimitTransitionRegionWidth=0.1  LowerLimitTransitionRegionWidthUnits=deg  UpperLimitSpecify=off  UpperLimitBound=90  UpperLimitBoundUnits=deg  UpperLimitStiffness=1e4  UpperLimitStiffnessUnits=N*m/deg  UpperLimitDamping=10  UpperLimitDampingUnits=N*m/(deg/s)  UpperLimitTransitionRegionWidth=0.1  UpperLimitTransitionRegionWidthUnits=deg  TorqueActuationMode=ComputedTorque  MotionActuationMode=InputMotion  SensePosition=off  SenseVelocity=off  SenseAcceleration=off  SenseTorqueForce=off  SenseLowerLimitTorqueForce=off  SenseUpperLimitTorqueForce=off
  Slew Drive : Subsystem  AncestorBlock=WormAndGearConstraintLibrary/Slew Drive  mask(Slew Drive){wormLeadAngle=slewdrive.wormLeadAngle, wormLength=slewdrive.wormLength, gearOuterRadius=slewdrive.gearOuterRadius, gearInnerRadius=slewdrive.gearInnerRadius, gearExposedRadius=slewdrive.gearExposedRadius, ratio=slewdrive.ratio, housingThickness=slewdrive.housingThickness, bWormRevolute=slewdrive.wormRevoluteDamping, wormRho=slewdrive.wormDensity, gearRho=slewdrive.gearDensity, housingRho=slewdrive.housingDensity, wormColor=slewdrive.wormColor, gearColor=slewdrive.gearColor, housingColor=slewdrive.housingColor, housingOpacity=slewdrive.housingOpacity}
      mask prompts: wormLeadAngle "Worm Lead Angle (deg)"; wormLength "Worm Length (m)"; gearOuterRadius "Gear Outer Radius (m)"; gearInnerRadius "Gear Inner Radius (m)"; gearExposedRadius "Gear Exposed Radius (m)"; ratio "Ratio (Ng / Nw)"; housingThickness "Housing Thickness (m)"; bWormRevolute "Worm Revolute Damping (Nm/(deg/s))"; wormRho "Worm Density (kg/m^3)"; gearRho "Gear Density (kg/m^3)"; housingRho "Housing Density (kg/m3)"; wormColor "Worm Color [r g b]"; gearColor "Gear Color [r g b]"; housingColor "Housing Color [r g b]"; housingOpacity "Housing Opacity"
      mask help:
      | This block models the slew drive of the solar tracker.
      |
      | Port B corresponds to the base face of the housing aligned with the gear axis. Port T corresponds to the center of the top face of the gear.
      |
      | Input port q specifies the motion actuation signal of the gear revolute. Output port w corresponds to the angular velocity of the worm revolute. Output port t corresponds to the automatically computed actuation torque at the worm revolute necessary to achieve the desired motion signal of the gear revolute.
      mask init: same as WormAndGearConstraint0x5B10x5D/Solar Array/Solar Tracker1/Slew Drive
      settings: LibrarySourceBlock=sm_solar_tracker_lib/Slew Drive
      mask DialogControl Tab1 Prompt: Dimensions
      mask DialogControl Tab2 Prompt: Internal Mechanics
      mask DialogControl Tab3 Prompt: Material Properties
      mask Display:
      | image(fullfile('WormAndGearConstraintSupport','Images','SlewDrive.png'));
      | port_label('lconn',1,'B');
      | port_label('lconn',2,'q');
      | port_label('rconn',1,'T');
      | port_label('rconn',2,'w');
      | port_label('rconn',3,'t');
  Solar Panel Assembly : Subsystem
      mask Display:
      | image(fullfile('WormAndGearConstraintSupport','Images','SolarPanel.png'));
      | port_label('lconn',1,'H');
  Support : Subsystem  AncestorBlock=WormAndGearConstraintLibrary/Support  mask(Support){columnRadius=support.columnRadius, columnThickness=support.columnThickness, columnHeight=support.columnHeight, baseWidth=support.baseWidth, baseThickness=support.baseThickness, rho=support.density, color=support.color}
      mask prompts: columnRadius "Column Radius (m)"; columnThickness "Column Thickness (m)"; columnHeight "Column Height (m)"; baseWidth "Base Width (m)"; baseThickness "Base Thickness (m)"; rho "Density (kg/m^3)"; color "Color [r g b]"
      mask help:
      | This block models the support for the solar tracker.
      |
      | Port B corresponds to the center of the base face. Port T corresponds to the center of the top face of the column.
      mask init: same as WormAndGearConstraint0x5B10x5D/Solar Array/Solar Tracker1/Support
      settings: LibrarySourceBlock=sm_solar_tracker_lib/Support
      mask DialogControl Tab1 Prompt: Dimensions
      mask DialogControl Tab2 Prompt: Material Properties
      mask Display:
      | image(fullfile('WormAndGearConstraintSupport','Images','Support.png'));
      | port_label('lconn',1,'B');
      | port_label('rconn',1,'T');
  B : PMIOPort  Side=Left
  y : PMIOPort  Port=2  Side=Left
  p : PMIOPort  Port=3  Side=Left
  w : PMIOPort  Port=4  Side=Right
  t : PMIOPort  Port=5  Side=Right
  connections:
  Support/LConn1 -- B/RConn1
  Support/RConn1 -- Slew Drive/LConn1
  Drive Connection/LConn1 -- Slew Drive/RConn1
  Panel Revolute/LConn1 -- Drive Connection/RConn1
  w/RConn1 -- Slew Drive/RConn2
  Slew Drive/LConn2 -- y/RConn1
  Panel Revolute/LConn2 -- p/RConn1
  Panel Revolute/RConn1 -- Solar Panel Assembly/LConn1
  t/RConn1 -- Slew Drive/RConn3

== system WormAndGearConstraint0x5B10x5D/Solar Array/Solar Tracker1/Drive Connection ==
  Bracket : Subsystem  AncestorBlock=WormAndGearConstraintLibrary/Single Bracket  mask(Single Bracket){height=bracketWidth, width=bracketWidth, thickness=bracketThickness, holeOffset=holeOffset, holeRadius=holeRadius, rho=rho, color=color}
      mask prompts: height "Height (m)"; width "Width (m)"; thickness "Thickness (m)"; holeOffset "Hole Offset (m)"; holeRadius "Hole Radius (m)"; rho "Density (kg/m^3)"; color "Color [r g b]"
      mask help:
      | This block models a bracket element.
      |
      | Port B corresponds to the center point of the base face. Port H corresponds to the center of the hole.
      mask DialogControl Tab1 Prompt: Dimensions
      mask DialogControl Tab2 Prompt: Material Properties
      mask Display:
      | image(fullfile('WormAndGearConstraintSupport','Images','SingleBracket.png'));
      | port_label('lconn',1,'B');
      | port_label('rconn',1,'H');
  Bracket Base : sm_lib/Body Elements/Cylindrical Solid  CylinderRadius=baseRadius  CylinderRadiusUnits=m  CylinderLength=baseThickness  CylinderLengthUnits=m  ExportEntireGeometry=off  InertiaType=CalculateFromGeometry  BasedOnType=Density  Density=rho  DensityUnits=kg/m^3  Mass=1  MassUnits=kg  CenterOfMass=[0 0 0]  CenterOfMassUnits=m  MomentsOfInertia=[1 1 1]  MomentsOfInertiaUnits=kg*m^2  ProductsOfInertia=[1 1 1]  ProductsOfInertiaUnits=kg*m^2  GraphicType=FromGeometry  MarkerShape=Sphere  MarkerSize=10  GraphicVisPropType=SimpleVisualProperties  GraphicDiffuseColor=color  GraphicOpacity=1.0  GraphicSpecularColor=[0.5 0.5 0.5 1.0]  GraphicAmbientColor=[0.15 0.15 0.15 1.0]  GraphicEmissiveColor=[0.0 0.0 0.0 1.0]  GraphicShininess=75  DoExposeReferenceFrame=off  SerializedFrames=<Frames><Frame><Id>Frame1</Id><Value><Name>T</Name><Origin><Source>GeometricFeature</Source><FeatureName>top surface</FeatureName></Origin><PrimaryAxis><DefinedDirection>+Z</DefinedDirection><Source>ReferenceFrame</Source><SourceDirection>+Z</SourceDirection><FeatureName></FeatureName></PrimaryAxis><SecondaryAxis><DefinedDirection>+X</DefinedDirection><Source>ReferenceFrame</Source><SourceDirection>-Y</SourceDirection><FeatureName></FeatureName></SecondaryAxis></Value></Frame><Frame><Id>Frame2</Id><Value><Name>B</Name><Origin><Source>GeometricFeature</Source><FeatureName>bottom surface</FeatureName></Origin><PrimaryAxis><DefinedDirection>+Z</DefinedDirection><Source>ReferenceFrame</Source><SourceDirection>+Z</SourceDirection><FeatureName></FeatureName></PrimaryAxis><SecondaryAxis><DefinedDirection>+X</DefinedDirection><Source>ReferenceFrame</Source><SourceDirection>+X</SourceDirection><FeatureName></FeatureName></SecondaryAxis></Value></Frame></Frames>
  Drive Connection : Subsystem  AncestorBlock=WormAndGearConstraintLibrary/Hollow Cylinder  mask(Hollow Cylinder){outerRadius=connRadius, thickness=connThickness, length=connLength, rho=rho, color=color}
      mask prompts: outerRadius "Outer Radius (m)"; thickness "Thickness (m)"; length "Length (m)"; rho "Density (kg/m^3)"; color "Color [r g b]"
      mask help:
      | This block models a hollow cylinder element.
      |
      | Port L corresponds to the left-hand end of the cylinder. Port R corresponds to the right-hand end of the cylinder.
      mask init:
      | innerRadius = outerRadius - thickness;
      | 
      | halfLength = 0.5*length;
      | 
      | crossSection = [...
      |   innerRadius -halfLength;...
      |   outerRadius -halfLength;...
      |   outerRadius  halfLength;...
      |   innerRadius  halfLength];
      mask DialogControl Tab1 Prompt: Dimensions
      mask DialogControl Tab2 Prompt: Material Properties
      mask Display:
      | image(fullfile('WormAndGearConstraintSupport','Images','HollowCylinder.png'));
      | port_label('lconn',1,'L');
      | port_label('rconn',1,'R');
  B : PMIOPort  Side=Left
  H : PMIOPort  Port=2  Side=Right
  connections:
  Drive Connection/LConn1 -- B/RConn1
  Drive Connection/RConn1 -- Bracket Base/RConn1
  Bracket Base/LConn1 -- Bracket/LConn1
  H/RConn1 -- Bracket/RConn1
